simulink model "dbap"  (Simulink 10.1)
settings: Solver=ode8  StartTime=0.0  StopTime=100  RelTol=1e-3
libraries: dsparch4 x2
settings Model: Creator=iba  LastModifiedBy=iba
settings DataIOCC: SaveFormat=Dataset  SaveOutput=off  SignalLogging=off  SaveTime=off  ReturnWorkspaceOutputs=on
settings OptimizationCC: DefaultParameterBehavior=Inlined  RollThreshold=2  LifeSpan=auto
settings DebuggingCC: AlgebraicLoopMsg=error  UnderspecifiedInitializationDetection=Simplified  MergeDetectMultiDrivingBlocksExec=error  SFUnexpectedBacktrackingDiag=error  SFNoUnconditionalDefaultTransitionDiag=error  SFExecutionAtInitializationDiag=warning  ArithmeticOperatorsInVariantConditions=error
settings HardwareCC: ProdBitPerPointer=64  ProdBitPerSizeT=64  ProdBitPerPtrDiffT=64  ProdLargestAtomicFloat=Float  ProdIntDivRoundTo=Zero  ProdEndianess=LittleEndian  ProdWordSize=64  ProdHWDeviceType=Intel->x86-64 (Windows64)
settings ModelReferenceCC: PropagateSignalLabelsOutOfModel=on
settings SFSimCC: SimUseLocalCustomCode=on  CustomCodeUndefinedFunction=FilterOut
settings RTWCC: RTWUseLocalCustomCode=on
settings CodeAppCC: StateflowObjectComments=off
settings GRTTargetCC: TargetLangStandard=C99 (ISO)  CombineOutputUpdateFcns=on  GRTInterface=off
settings ConfigComp: CovMetricSettings=dwe  CovHtmlReporting=off  CovSaveCumulativeToWorkspaceVar=off  CovSaveSingleToWorkspaceVar=off  CovExternalEMLEnable=on

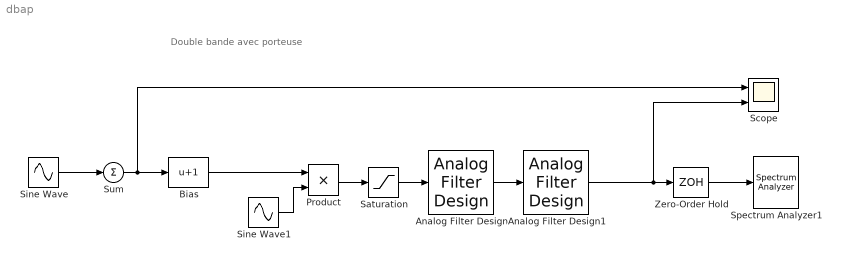
== system dbap ==
  note: Double bande avec porteuse
  Analog Filter Design : dsparch4/Analog Filter Design  method=Butterworth  filttype=Lowpass  N=4  Wlo=5  Whi=80  Rp=2  Rs=40
  Analog Filter Design1 : dsparch4/Analog Filter Design  method=Butterworth  filttype=Highpass  N=4  Wlo=0.1  Whi=80  Rp=2  Rs=40
  Bias : Bias  Bias=1
  Product : Product
  Saturation : Saturate  UpperLimit=100  LowerLimit=0
  Scope : Scope  NumInputPorts=2
  Sine Wave : Sin  Amplitude=linspace(0.15,0.1,9)  Frequency=(1:0.5:5)  SampleTime=0.1
  Sine Wave1 : Sin  Frequency=25  SampleTime=0.1
  Spectrum Analyzer1 : SpectrumAnalyzer
  Sum : Sum  Inputs=+
  Zero-Order Hold : ZeroOrderHold  SampleTime=0.2
  wires:
  Sine Wave/1 -> Sum/1
  Sum/1 -> Scope/1, Bias/1
  Sine Wave1/1 -> Product/2
  Product/1 -> Saturation/1
  Bias/1 -> Product/1
  Zero-Order Hold/1 -> Spectrum Analyzer1/1
  Saturation/1 -> Analog Filter Design/1
  Analog Filter Design/1 -> Analog Filter Design1/1
  Analog Filter Design1/1 -> Scope/2, Zero-Order Hold/1
